simulink model "Position_Controller_Phy"  (R2022a)
settings: Solver=VariableStepAuto  StartTime=0.0  StopTime=20  RelTol=1e-3
undefined symbols (not defined in the file): A_0, A_0k, d, F_0, F_0k, g, Gi_s, Gp_s, ktd_s, m, M, P_0, P_0k, PI, Ts
settings Model: Creator=DELL  LastModifiedBy=DELL

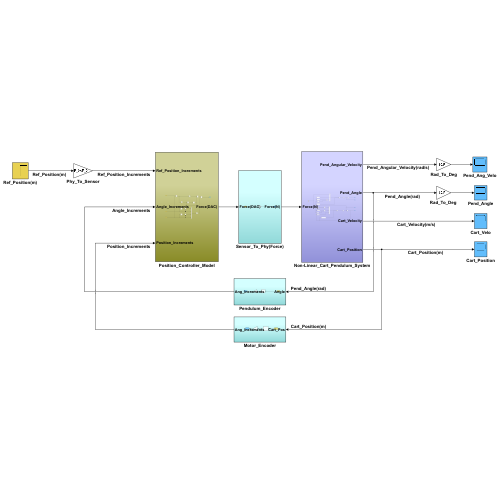
[thumbnail: Simulink's stored preview of the top-level diagram]
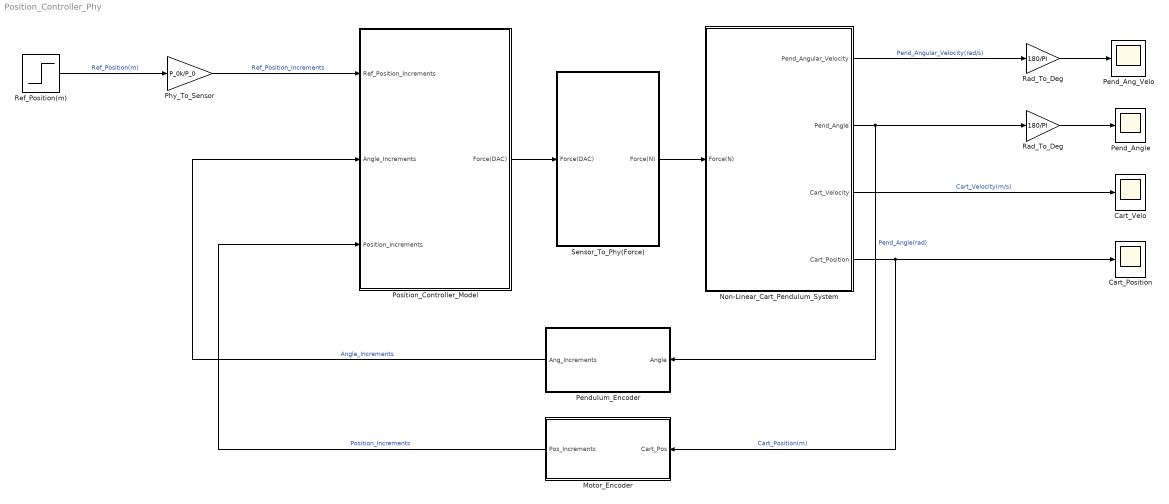
== system Position_Controller_Phy ==
  Cart_Position : Scope
  Cart_Velo : Scope
  Motor_Encoder : Subsystem
  Non-Linear_Cart_Pendulum_System : Subsystem
  Pend_Ang_Velo : Scope
  Pend_Angle : Scope
  Pendulum_Encoder : Subsystem
  Phy_To_Sensor : Gain  Gain=P_0k/P_0
  Position_Controller_Model : Subsystem
  Rad_To_Deg : Gain  Gain=180/PI
  "Rad_To_Deg " : Gain  Gain=180/PI
  Ref_Position(m) : Step  SampleTime=Ts
  Sensor_To_Phy(Force) : Subsystem
  wires:
  Ref_Position(m)/1 -> Phy_To_Sensor/1  "Ref_Position(m)"
  Non-Linear_Cart_Pendulum_System/3(Cart_Velocity) -> Cart_Velo/1  "Cart_Velocity(m/s)"
  Non-Linear_Cart_Pendulum_System/4(Cart_Position) -> Motor_Encoder/1(Cart_Pos), Cart_Position/1  "Cart_Position(m)"
  Non-Linear_Cart_Pendulum_System/1(Pend_Angular_Velocity) -> Rad_To_Deg/1  "Pend_Angular_Velocity(rad/s)"
  Phy_To_Sensor/1 -> Position_Controller_Model/1(Ref_Position_Increments)  "Ref_Position_Increments"
  Position_Controller_Model/1(Force(DAC)) -> Sensor_To_Phy(Force)/1(Force(DAC))
  Sensor_To_Phy(Force)/1(Force(N)) -> Non-Linear_Cart_Pendulum_System/1(Force(N))
  Non-Linear_Cart_Pendulum_System/2(Pend_Angle) -> Pendulum_Encoder/1(Angle), "Rad_To_Deg "/1  "Pend_Angle(rad)"
  Pendulum_Encoder/1(Ang_Increments) -> Position_Controller_Model/2(Angle_Increments)  "Angle_Increments"
  Motor_Encoder/1(Pos_Increments) -> Position_Controller_Model/3(Position_Increments)  "Position_Increments"
  "Rad_To_Deg "/1 -> Pend_Angle/1
  Rad_To_Deg/1 -> Pend_Ang_Velo/1

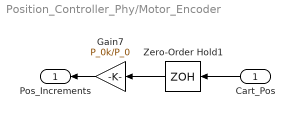
== system Position_Controller_Phy/Motor_Encoder ==
  Cart_Pos : Inport
  Gain7 : Gain  Gain=P_0k/P_0
  Zero-Order Hold1 : ZeroOrderHold  SampleTime=Ts
  Pos_Increments : Outport
  wires:
  Gain7/1 -> Pos_Increments/1
  Zero-Order Hold1/1 -> Gain7/1
  Cart_Pos/1 -> Zero-Order Hold1/1

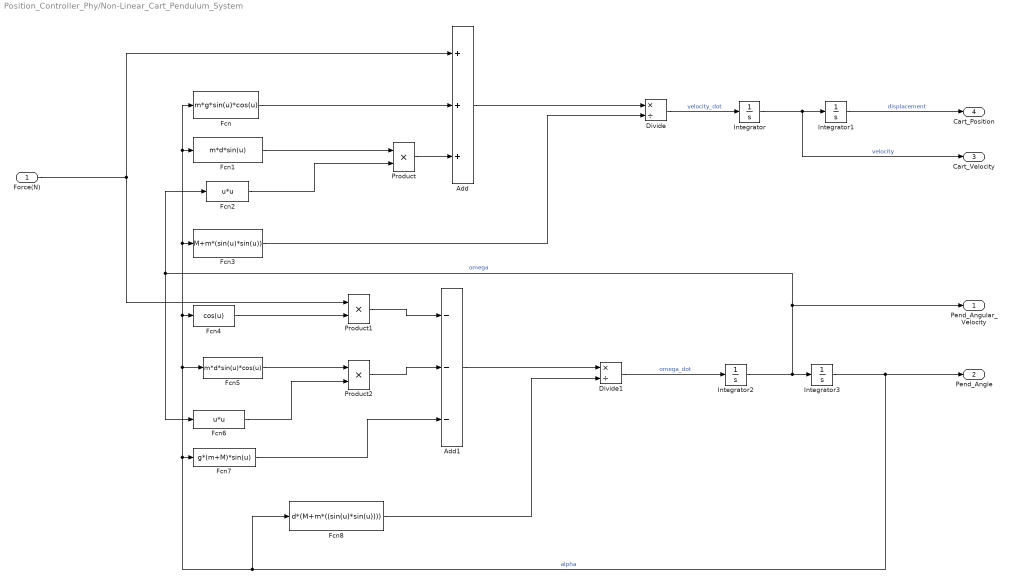
== system Position_Controller_Phy/Non-Linear_Cart_Pendulum_System ==
  Force(N) : Inport
  Add : Sum  Inputs=+++
  Add1 : Sum  Inputs=---
  Divide : Product  Inputs=*/
  Divide1 : Product  Inputs=*/
  Fcn : Fcn  Expr=m*g*sin(u)*cos(u)
  Fcn1 : Fcn  Expr=m*d*sin(u)
  Fcn2 : Fcn  Expr=u*u
  Fcn3 : Fcn  Expr=M+m*(sin(u)*sin(u))
  Fcn4 : Fcn  Expr=cos(u)
  Fcn5 : Fcn  Expr=m*d*sin(u)*cos(u)
  Fcn6 : Fcn  Expr=u*u
  Fcn7 : Fcn  Expr=g*(m+M)*sin(u)
  Fcn8 : Fcn  Expr=d*(M+m*((sin(u)*sin(u))))
  Integrator{,1..3} (4 alike) : Integrator
  Product : Product
  Product1 : Product
  Product2 : Product
  Pend_Angular_Velocity : Outport  VectorParamsAs1DForOutWhenUnconnected=off
  Pend_Angle : Outport  Port=2  VectorParamsAs1DForOutWhenUnconnected=off
  Cart_Velocity : Outport  Port=3  VectorParamsAs1DForOutWhenUnconnected=off
  Cart_Position : Outport  Port=4  VectorParamsAs1DForOutWhenUnconnected=off
  wires:
  Add/1 -> Divide/1
  Integrator2/1 -> Integrator3/1, Pend_Angular_Velocity/1, Fcn2/1, Fcn6/1  "omega"
  Fcn1/1 -> Product/1
  Integrator1/1 -> Cart_Position/1  "displacement"
  Fcn6/1 -> Product2/2
  Product/1 -> Add/3
  Fcn2/1 -> Product/2
  Fcn4/1 -> Product1/2
  Fcn/1 -> Add/2
  Integrator3/1 -> Pend_Angle/1, Fcn8/1, Fcn7/1, Fcn5/1, Fcn4/1, Fcn/1, Fcn1/1, Fcn3/1  "alpha"
  Divide/1 -> Integrator/1  "velocity_dot"
  Fcn3/1 -> Divide/2
  Product2/1 -> Add1/2
  Add1/1 -> Divide1/1
  Fcn5/1 -> Product2/1
  Product1/1 -> Add1/1
  Fcn8/1 -> Divide1/2
  Fcn7/1 -> Add1/3
  Force(N)/1 -> Add/1, Product1/1
  Integrator/1 -> Integrator1/1, Cart_Velocity/1  "velocity"
  Divide1/1 -> Integrator2/1  "omega_dot"

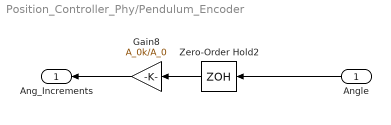
== system Position_Controller_Phy/Pendulum_Encoder ==
  Angle : Inport
  Gain8 : Gain  Gain=A_0k/A_0
  Zero-Order Hold2 : ZeroOrderHold  SampleTime=Ts
  Ang_Increments : Outport
  wires:
  Zero-Order Hold2/1 -> Gain8/1
  Angle/1 -> Zero-Order Hold2/1
  Gain8/1 -> Ang_Increments/1

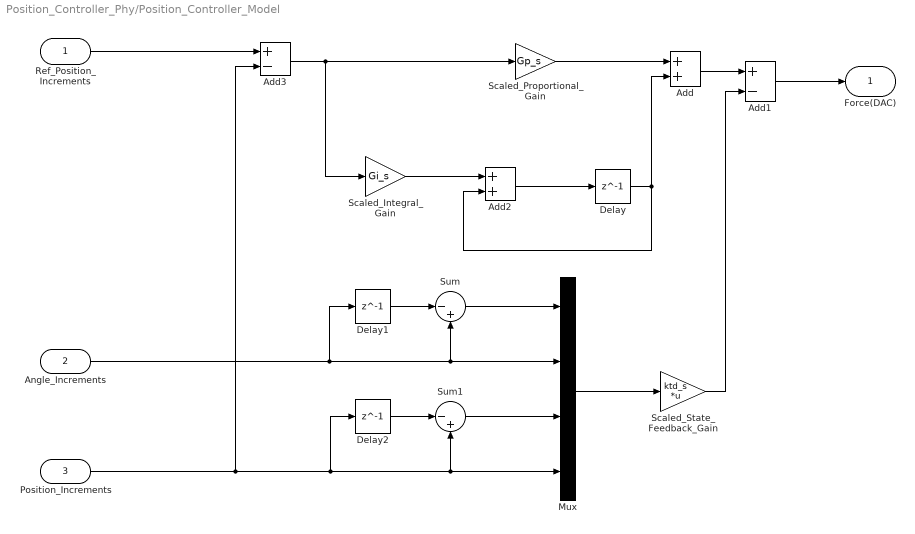
== system Position_Controller_Phy/Position_Controller_Model ==
  Ref_Position_Increments : Inport
  Angle_Increments : Inport  Port=2
  Position_Increments : Inport  Port=3
  Add : Sum
  Add1 : Sum  Inputs=+-
  Add2 : Sum
  Add3 : Sum  Inputs=+-
  Delay : Delay  DelayLength=1  SampleTime=Ts
  Delay1 : Delay  DelayLength=1  SampleTime=Ts
  Delay2 : Delay  DelayLength=1  SampleTime=Ts
  Mux : Mux
  Scaled_Integral_Gain : Gain  Gain=Gi_s
  Scaled_Proportional_Gain : Gain  Gain=Gp_s
  Scaled_State_Feedback_Gain : Gain  Gain=ktd_s  Multiplication=Matrix(K*u) (u vector)
  Sum : Sum  Inputs=|-+
  Sum1 : Sum  Inputs=|-+
  Force(DAC) : Outport
  wires:
  Add2/1 -> Delay/1
  Scaled_Integral_Gain/1 -> Add2/1
  Add/1 -> Add1/1
  Scaled_Proportional_Gain/1 -> Add/1
  Delay/1 -> Add/2, Add2/2
  Add3/1 -> Scaled_Integral_Gain/1, Scaled_Proportional_Gain/1
  Add1/1 -> Force(DAC)/1
  Ref_Position_Increments/1 -> Add3/1
  Angle_Increments/1 -> Sum/2, Mux/2, Delay1/1
  Delay1/1 -> Sum/1
  Sum/1 -> Mux/1
  Delay2/1 -> Sum1/1
  Sum1/1 -> Mux/3
  Position_Increments/1 -> Add3/2, Delay2/1, Sum1/2, Mux/4
  Mux/1 -> Scaled_State_Feedback_Gain/1
  Scaled_State_Feedback_Gain/1 -> Add1/2

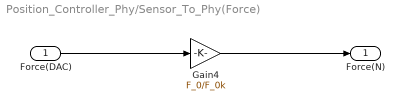
== system Position_Controller_Phy/Sensor_To_Phy(Force) ==
  Force(DAC) : Inport
  Gain4 : Gain  Gain=F_0/F_0k
  Force(N) : Outport
  wires:
  Force(DAC)/1 -> Gain4/1
  Gain4/1 -> Force(N)/1
